simulink model "simulation__"  (R2021a)
settings: Solver=ode14x  StartTime=0.0  StopTime=40  FixedStep=0.01  RelTol=1e-3
values from neighbouring files (symbols this model uses):
  Rep = 1.655    [coefficients.m]
  Rev = 0.04    [coefficients.m]
  Rla = 2.5e-3    (= 0.0025)    [coefficients.m]
  Rpa = 0.023    [coefficients.m]
  Rpp = 0.091    [coefficients.m]
  Rpv = 0.0056    [coefficients.m]
  Rra = 2.5e-3    (= 0.0025)    [coefficients.m]
  Rsa = 0.06    [coefficients.m]
  Rsp = 2.491    [coefficients.m]
  Rsv = 0.038    [coefficients.m]
  Vulv = 16.77    [coefficients.m]
  Vurv = 40.8    [coefficients.m]
libraries: ee_lib x26, fl_lib x20, nesl_utility x11
settings Model: Creator=Buyson  LastModifiedBy=Buyson

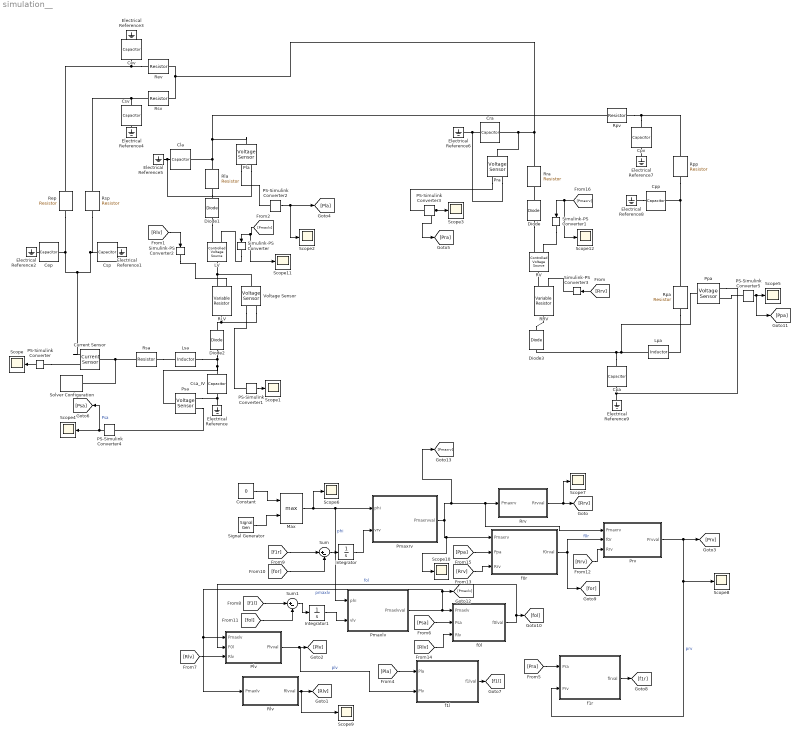
== system simulation__ ==
  Cep : ee_lib/Passive/Capacitor  cap_option=0  c=Cep F  Cvec=[1e-05, 1e-06] F  Vvec=[0, 10] V  CV_table_symmetry=1  f_vec=[1, 10] kHz  DFext_vec=[.8, 1.2]  C_tol=5  enable_C_tol=0  tol_distribution=1  nSigma=4  r=1e-6 Ohm  g=0 1/Ohm  averaging_period=0 s  enable_operating_limits=0  operating_limit_action=2  max_working_voltage_range=[-25, 25] V  power_rating=1 W  enable_faults=0  fault_action=1  Cscale_faulted=100  R_faulted=1e-3 Ohm  G_faulted=0 1/Ohm  tau_fault=1e-3 s  enable_temporal_fault=0  t_fault=1 s  enable_behavioral_fault=0  max_permissible_voltage_range=[-100, 100] V  t_fail_on_voltage=1 s  i_specify=off  i_priority=None  i=0 A  i_nominal_specify=off  i_nominal_unit=A  i_nominal_value=1  v_specify=off  v_priority=None  v=0 V  v_nominal_specify=off  v_nominal_unit=V  v_nominal_value=1  vc_specify=on  vc_priority=High  vc=Cep_IV V  vc_nominal_specify=off  vc_nominal_unit=V  vc_nominal_value=1
  Cev : ee_lib/Passive/Capacitor  cap_option=0  c=Cev F  Cvec=[1e-05, 1e-06] F  Vvec=[0, 10] V  CV_table_symmetry=1  f_vec=[1, 10] kHz  DFext_vec=[.8, 1.2]  C_tol=5  enable_C_tol=0  tol_distribution=1  nSigma=4  r=1e-6 Ohm  g=0 1/Ohm  averaging_period=0 s  enable_operating_limits=0  operating_limit_action=2  max_working_voltage_range=[-25, 25] V  power_rating=1 W  enable_faults=0  fault_action=1  Cscale_faulted=100  R_faulted=1e-3 Ohm  G_faulted=0 1/Ohm  tau_fault=1e-3 s  enable_temporal_fault=0  t_fault=1 s  enable_behavioral_fault=0  max_permissible_voltage_range=[-100, 100] V  t_fail_on_voltage=1 s  i_specify=off  i_priority=None  i=0 A  i_nominal_specify=off  i_nominal_unit=A  i_nominal_value=1  v_specify=off  v_priority=None  v=0 V  v_nominal_specify=off  v_nominal_unit=V  v_nominal_value=1  vc_specify=on  vc_priority=High  vc=Cev_IV V  vc_nominal_specify=off  vc_nominal_unit=V  vc_nominal_value=1
  Cla : ee_lib/Passive/Capacitor  cap_option=0  c=Cla F  Cvec=[1e-05, 1e-06] F  Vvec=[0, 10] V  CV_table_symmetry=1  f_vec=[1, 10] kHz  DFext_vec=[.8, 1.2]  C_tol=5  enable_C_tol=0  tol_distribution=1  nSigma=4  r=1e-6 Ohm  g=0 1/Ohm  averaging_period=0 s  enable_operating_limits=0  operating_limit_action=2  max_working_voltage_range=[-25, 25] V  power_rating=1 W  enable_faults=0  fault_action=1  Cscale_faulted=100  R_faulted=1e-3 Ohm  G_faulted=0 1/Ohm  tau_fault=1e-3 s  enable_temporal_fault=0  t_fault=1 s  enable_behavioral_fault=0  max_permissible_voltage_range=[-100, 100] V  t_fail_on_voltage=1 s  i_specify=off  i_priority=None  i=0 A  i_nominal_specify=off  i_nominal_unit=A  i_nominal_value=1  v_specify=off  v_priority=None  v=0 V  v_nominal_specify=off  v_nominal_unit=V  v_nominal_value=1  vc_specify=on  vc_priority=High  vc=Cla_IV V  vc_nominal_specify=off  vc_nominal_unit=V  vc_nominal_value=1
  Constant : Constant  Value=0
  Cpa : ee_lib/Passive/Capacitor  cap_option=0  c=Cpa F  Cvec=[1e-05, 1e-06] F  Vvec=[0, 10] V  CV_table_symmetry=1  f_vec=[1, 10] kHz  DFext_vec=[.8, 1.2]  C_tol=5  enable_C_tol=0  tol_distribution=1  nSigma=4  r=1e-6 Ohm  g=0 1/Ohm  averaging_period=0 s  enable_operating_limits=0  operating_limit_action=2  max_working_voltage_range=[-25, 25] V  power_rating=1 W  enable_faults=0  fault_action=1  Cscale_faulted=100  R_faulted=1e-3 Ohm  G_faulted=0 1/Ohm  tau_fault=1e-3 s  enable_temporal_fault=0  t_fault=1 s  enable_behavioral_fault=0  max_permissible_voltage_range=[-100, 100] V  t_fail_on_voltage=1 s  i_specify=off  i_priority=None  i=0 A  i_nominal_specify=off  i_nominal_unit=A  i_nominal_value=1  v_specify=off  v_priority=None  v=0 V  v_nominal_specify=off  v_nominal_unit=V  v_nominal_value=1  vc_specify=on  vc_priority=High  vc=Cpa_IV V  vc_nominal_specify=off  vc_nominal_unit=V  vc_nominal_value=1
  Cpp : ee_lib/Passive/Capacitor  cap_option=0  c=Cpp F  Cvec=[1e-05, 1e-06] F  Vvec=[0, 10] V  CV_table_symmetry=1  f_vec=[1, 10] kHz  DFext_vec=[.8, 1.2]  C_tol=5  enable_C_tol=0  tol_distribution=1  nSigma=4  r=1e-6 Ohm  g=0 1/Ohm  averaging_period=0 s  enable_operating_limits=0  operating_limit_action=2  max_working_voltage_range=[-25, 25] V  power_rating=1 W  enable_faults=0  fault_action=1  Cscale_faulted=100  R_faulted=1e-3 Ohm  G_faulted=0 1/Ohm  tau_fault=1e-3 s  enable_temporal_fault=0  t_fault=1 s  enable_behavioral_fault=0  max_permissible_voltage_range=[-100, 100] V  t_fail_on_voltage=1 s  i_specify=off  i_priority=None  i=0 A  i_nominal_specify=off  i_nominal_unit=A  i_nominal_value=1  v_specify=off  v_priority=None  v=0 V  v_nominal_specify=off  v_nominal_unit=V  v_nominal_value=1  vc_specify=on  vc_priority=High  vc=Cpp_IV V  vc_nominal_specify=off  vc_nominal_unit=V  vc_nominal_value=1
  Cpv : ee_lib/Passive/Capacitor  cap_option=0  c=Cpv F  Cvec=[1e-05, 1e-06] F  Vvec=[0, 10] V  CV_table_symmetry=1  f_vec=[1, 10] kHz  DFext_vec=[.8, 1.2]  C_tol=5  enable_C_tol=0  tol_distribution=1  nSigma=4  r=1e-6 Ohm  g=0 1/Ohm  averaging_period=0 s  enable_operating_limits=0  operating_limit_action=2  max_working_voltage_range=[-25, 25] V  power_rating=1 W  enable_faults=0  fault_action=1  Cscale_faulted=100  R_faulted=1e-3 Ohm  G_faulted=0 1/Ohm  tau_fault=1e-3 s  enable_temporal_fault=0  t_fault=1 s  enable_behavioral_fault=0  max_permissible_voltage_range=[-100, 100] V  t_fail_on_voltage=1 s  i_specify=off  i_priority=None  i=0 A  i_nominal_specify=off  i_nominal_unit=A  i_nominal_value=1  v_specify=off  v_priority=None  v=0 V  v_nominal_specify=off  v_nominal_unit=V  v_nominal_value=1  vc_specify=on  vc_priority=High  vc=Cpv_IV V  vc_nominal_specify=off  vc_nominal_unit=V  vc_nominal_value=1
  Cra : ee_lib/Passive/Capacitor  cap_option=0  c=Cra F  Cvec=[1e-05, 1e-06] F  Vvec=[0, 10] V  CV_table_symmetry=1  f_vec=[1, 10] kHz  DFext_vec=[.8, 1.2]  C_tol=5  enable_C_tol=0  tol_distribution=1  nSigma=4  r=1e-6 Ohm  g=0 1/Ohm  averaging_period=0 s  enable_operating_limits=0  operating_limit_action=2  max_working_voltage_range=[-25, 25] V  power_rating=1 W  enable_faults=0  fault_action=1  Cscale_faulted=100  R_faulted=1e-3 Ohm  G_faulted=0 1/Ohm  tau_fault=1e-3 s  enable_temporal_fault=0  t_fault=1 s  enable_behavioral_fault=0  max_permissible_voltage_range=[-100, 100] V  t_fail_on_voltage=1 s  i_specify=off  i_priority=None  i=0 A  i_nominal_specify=off  i_nominal_unit=A  i_nominal_value=1  v_specify=off  v_priority=None  v=0 V  v_nominal_specify=off  v_nominal_unit=V  v_nominal_value=1  vc_specify=on  vc_priority=High  vc=Cra_IV V  vc_nominal_specify=off  vc_nominal_unit=V  vc_nominal_value=1
  Csa_IV : ee_lib/Passive/Capacitor  cap_option=0  c=Csa F  Cvec=[1e-05, 1e-06] F  Vvec=[0, 10] V  CV_table_symmetry=1  f_vec=[1, 10] kHz  DFext_vec=[.8, 1.2]  C_tol=5  enable_C_tol=0  tol_distribution=1  nSigma=4  r=1e-6 Ohm  g=0 1/Ohm  averaging_period=0 s  enable_operating_limits=0  operating_limit_action=2  max_working_voltage_range=[-25, 25] V  power_rating=1 W  enable_faults=0  fault_action=1  Cscale_faulted=100  R_faulted=1e-3 Ohm  G_faulted=0 1/Ohm  tau_fault=1e-3 s  enable_temporal_fault=0  t_fault=1 s  enable_behavioral_fault=0  max_permissible_voltage_range=[-100, 100] V  t_fail_on_voltage=1 s  i_specify=off  i_priority=None  i=0 A  i_nominal_specify=off  i_nominal_unit=A  i_nominal_value=1  v_specify=off  v_priority=None  v=0 V  v_nominal_specify=off  v_nominal_unit=V  v_nominal_value=1  vc_specify=on  vc_priority=High  vc=Csa_IV V  vc_nominal_specify=off  vc_nominal_unit=V  vc_nominal_value=1
  Csp : ee_lib/Passive/Capacitor  cap_option=0  c=Csp F  Cvec=[1e-05, 1e-06] F  Vvec=[0, 10] V  CV_table_symmetry=1  f_vec=[1, 10] kHz  DFext_vec=[.8, 1.2]  C_tol=5  enable_C_tol=0  tol_distribution=1  nSigma=4  r=1e-6 Ohm  g=0 1/Ohm  averaging_period=0 s  enable_operating_limits=0  operating_limit_action=2  max_working_voltage_range=[-25, 25] V  power_rating=1 W  enable_faults=0  fault_action=1  Cscale_faulted=100  R_faulted=1e-3 Ohm  G_faulted=0 1/Ohm  tau_fault=1e-3 s  enable_temporal_fault=0  t_fault=1 s  enable_behavioral_fault=0  max_permissible_voltage_range=[-100, 100] V  t_fail_on_voltage=1 s  i_specify=off  i_priority=None  i=0 A  i_nominal_specify=off  i_nominal_unit=A  i_nominal_value=1  v_specify=off  v_priority=None  v=0 V  v_nominal_specify=off  v_nominal_unit=V  v_nominal_value=1  vc_specify=on  vc_priority=High  vc=Csp_IV V  vc_nominal_specify=off  vc_nominal_unit=V  vc_nominal_value=1
  Csv : ee_lib/Passive/Capacitor  cap_option=0  c=Csv F  Cvec=[1e-05, 1e-06] F  Vvec=[0, 10] V  CV_table_symmetry=1  f_vec=[1, 10] kHz  DFext_vec=[.8, 1.2]  C_tol=5  enable_C_tol=0  tol_distribution=1  nSigma=4  r=1e-6 Ohm  g=0 1/Ohm  averaging_period=0 s  enable_operating_limits=0  operating_limit_action=2  max_working_voltage_range=[-25, 25] V  power_rating=1 W  enable_faults=0  fault_action=1  Cscale_faulted=100  R_faulted=1e-3 Ohm  G_faulted=0 1/Ohm  tau_fault=1e-3 s  enable_temporal_fault=0  t_fault=1 s  enable_behavioral_fault=0  max_permissible_voltage_range=[-100, 100] V  t_fail_on_voltage=1 s  i_specify=off  i_priority=None  i=0 A  i_nominal_specify=off  i_nominal_unit=A  i_nominal_value=1  v_specify=off  v_priority=None  v=0 V  v_nominal_specify=off  v_nominal_unit=V  v_nominal_value=1  vc_specify=on  vc_priority=High  vc=Csv_IV V  vc_nominal_specify=off  vc_nominal_unit=V  vc_nominal_value=1
  Current Sensor : fl_lib/Electrical/Electrical Sensors/Current Sensor
  Diode{,1..3} (4 alike) : ee_lib/Semiconductors & Converters/Diode  ModelType=ee.enum.diode.modelType.pwl  IfMat=[.07, .12, .19, 1.75, 4.24, 7.32, 11.2; .16, .3, .72, 2.14, 4.02, 6.35, 9.12] A  TjVec=[25, 125] degC  VfVec=[.5, .7, .9, 1.3, 1.7, 2.1, 2.5] V  Vf=1e-4 V  Ron=1e-10 Ohm  Goff=1e-10 S  prmExp=ee.enum.diode.expParam.useTwo  I12=[.0137, .545] A  V12=[.6, .7] V  IS=1e-12 A  ec=1  I1=0.0137 A  V1=0.6 V  RS=0 Ohm  Tmeas=25 degC  N_series=1  N_parallel=1  Rz=0.3 Ohm  BV=inf V  C_param=ee.enum.diode.capParam.fixed  CJ=5 pF  CJ0=5 pF  VJ=1 V  Mgrad=0.5  Vvec=[.1, 10, 100] V  Cvec=[3.5, 1, .4] pF  FC=0.5  Q_param=ee.enum.diode.recoveryParam.off  iRM=-7.15 A  iF=4 A  didt=-750 A/us  trr_factor=3  trr=115 ns  Qrr=150 s*nA  TT=50 ns  tau=100 ns  T_param=ee.enum.diode.temperatureParam.off  IS_T2=1.25e-7 A  I1_T2=0.245 A  V1_T2=0.5 V  Tmeas2=125 degC  EG_param=ee.enum.diode.egapParam.material_si  EG=1.11 eV  XTI_param=ee.enum.diode.xtiParam.pn  XTI=3  dBVdT=0 V/K  enable_faults=ee.enum.faults.faultEnable.no  fault_action=ee.enum.faults.faultAction.none  fault_types=ee.enum.diode.faults.open  tau_fault=1e-3 s  IfMat_faulted=[.07, .12, .19, 1.75, 4.24, 7.32, 11.2; .16, .3, .72, 2.14, 4.02, 6.35, 9.12] A  VfVec_faulted=[.5, .7, .9, 1.3, 1.7, 2.1, 2.5] V  Ropen_faulted=1000 Ohm  Gshort_faulted=1000 1/Ohm  Vf_faulted=0.6 V  Ron_faulted=0.3 Ohm  Goff_faulted=1e-8 S  I12_faulted=[.0137, .545] A  V12_faulted=[.6, .7] V  IS_faulted=1e-12 A  ec_faulted=1  I1_faulted=0.0137 A  V1_faulted=0.6 V  RS_faulted=0 Ohm  Rz_faulted=0.3 Ohm  BV_faulted=inf V  Cscale_faulted=100  enable_temporal_fault=ee.enum.faults.faultEnable.no  t_fault=inf s  enable_behavioral_fault=ee.enum.faults.faultEnable.no  max_permissible_voltage=inf V  n_fail_on_voltage=1  max_permissible_current=inf A  t_fail_on_current=1 s  max_permissible_dVdt=inf V/s  Tdevice=25 degC  i_specify=off  i_priority=None  i=0 A  i_nominal_specify=off  i_nominal_unit=A  i_nominal_value=1  v_specify=on  v_priority=None  v=1e-4 V  v_nominal_specify=off  v_nominal_unit=V  v_nominal_value=1  i_diode_specify=off  i_diode_priority=None  i_diode=0 A  i_diode_nominal_specify=off  i_diode_nominal_unit=A  i_diode_nominal_value=1  v_diode_specify=off  v_diode_priority=None  v_diode=0 V  v_diode_nominal_specify=off  v_diode_nominal_unit=V  v_diode_nominal_value=1  i_capacitor_specify=off  i_capacitor_priority=None  i_capacitor=0 A  i_capacitor_nominal_specify=off  i_capacitor_nominal_unit=A  i_capacitor_nominal_value=1  v_capacitor_specify=off  v_capacitor_priority=None  v_capacitor=0 V  v_capacitor_nominal_specify=off  v_capacitor_nominal_unit=V  v_capacitor_nominal_value=1  power_dissipated_specify=off  power_dissipated_priority=None  power_dissipated=0 W  power_dissipated_nominal_specify=off  power_dissipated_nominal_unit=W  power_dissipated_nominal_value=1  max_permissible_temperature=inf K  t_fail_on_temperature=1 s  thermal_network_parameterization=ee.enum.thermalNetworkTopology.cauer  Rth=[0, 10] K/W  Rth_Foster=[4, 6] K/W  thermal_mass_parameterization=ee.enum.thermalNetwork.timeconstant  thermal_mass=[0, 1] J/K  thermal_mass_Foster=[1.5, 3] J/K  thermal_time_constant=[0, 10] s  thermal_time_constant_Foster=[6, 18] s  thermal_mass_initial_temperatures=[25, 25] degC
  Electrical Reference{,1..9} (10 alike) : fl_lib/Electrical/Electrical Elements/Electrical Reference
  Integrator : Integrator  InitialCondition=Vurv
  Integrator1 : Integrator  InitialCondition=Vulv
  LV : fl_lib/Electrical/Electrical Sources/Controlled Voltage Source
  Lpa : ee_lib/Passive/Inductor  l=Lpa H  L_tol=20  enable_L_tol=0  tol_distribution=1  nSigma=4  r=0 Ohm  g=1e-9 1/Ohm  enable_operating_limits=0  operating_limit_action=2  max_working_current=1 A  power_rating=1 W  enable_faults=0  fault_action=1  lambdaPercent=50  k_faulted=0.9999  turnsShort=0  openCct=0  groundShort=0  groundShortG=0 1/Ohm  tau_fault=1e-3 s  enable_temporal_fault=0  t_fault=1 s  enable_behavioral_fault=0  max_permissible_voltage=100 V  n_fail_on_voltage=1  max_permissible_current=1 A  t_fail_on_current=1 s  i_L_specify=off  i_L_priority=High  i_L=0 A  i_L_nominal_specify=off  i_L_nominal_unit=A  i_L_nominal_value=1
  Lsa : ee_lib/Passive/Inductor  l=Lsa H  L_tol=20  enable_L_tol=0  tol_distribution=1  nSigma=4  r=0 Ohm  g=1e-9 1/Ohm  enable_operating_limits=0  operating_limit_action=2  max_working_current=1 A  power_rating=1 W  enable_faults=0  fault_action=1  lambdaPercent=50  k_faulted=0.9999  turnsShort=0  openCct=0  groundShort=0  groundShortG=0 1/Ohm  tau_fault=1e-3 s  enable_temporal_fault=0  t_fault=1 s  enable_behavioral_fault=0  max_permissible_voltage=100 V  n_fail_on_voltage=1  max_permissible_current=1 A  t_fail_on_current=1 s  i_L_specify=off  i_L_priority=High  i_L=0 A  i_L_nominal_specify=off  i_L_nominal_unit=A  i_L_nominal_value=1
  Max : MinMax  Function=max  Inputs=2
  PS-Simulink Converter{,1..5} (6 alike) : nesl_utility/PS-Simulink Converter  PhysicalDomain=network_engine_domain  SubClassName=ps_output  LeftPortType=input  RightPortType=output  PseudoPeriodic=off  Frequencies=[]  Unit=inherit  AffineConversion=off
      settings: SourceProductBaseCode=PW,SS
  Pla : fl_lib/Electrical/Electrical Sensors/Voltage Sensor
  Plv : MATLAB Function  TreatAsAtomicUnit=on
  Pmaxlv : MATLAB Function  TreatAsAtomicUnit=on
  Pmaxrv : MATLAB Function  TreatAsAtomicUnit=on
  Ppa : fl_lib/Electrical/Electrical Sensors/Voltage Sensor
  Pra : fl_lib/Electrical/Electrical Sensors/Voltage Sensor
  Prv : MATLAB Function  TreatAsAtomicUnit=on
  Psa : fl_lib/Electrical/Electrical Sensors/Voltage Sensor
  RLV : fl_lib/Electrical/Electrical Elements/Variable Resistor  Rmin=0 Ohm  i_specify=off  i_priority=None  i=0 A  i_nominal_specify=off  i_nominal_unit=A  i_nominal_value=1  v_specify=off  v_priority=None  v=0 V  v_nominal_specify=off  v_nominal_unit=V  v_nominal_value=1
  RRV : fl_lib/Electrical/Electrical Elements/Variable Resistor  Rmin=0 Ohm  i_specify=off  i_priority=None  i=0 A  i_nominal_specify=off  i_nominal_unit=A  i_nominal_value=1  v_specify=off  v_priority=None  v=0 V  v_nominal_specify=off  v_nominal_unit=V  v_nominal_value=1
  RV : fl_lib/Electrical/Electrical Sources/Controlled Voltage Source
  Rep : ee_lib/Passive/Resistor  R=Rep Ohm  R_tol=5  enable_R_tol=0  tol_distribution=1  nSigma=4  enable_operating_limits=0  operating_limit_action=2  max_working_voltage=100 V  power_rating=1 W  enable_faults=0  fault_action=1  R_faulted=inf Ohm  enable_temporal_fault=0  t_fault=1 s  enable_behavioral_fault=0  max_permissible_current=1 A  t_fail_on_current=1 s  noise_mode=0  sample_time=1e-3 s  repeatability=1  auto_seed=3499211588  user_seed=0  Tdevice=25 degC  alpha=3.93e-3 1/K  Tmeas=25 degC  thermal_mass=100 J/K  power_derating_T1=70 degC  power_derating_T2=155 degC  operating_temperature_range_vec=[-50, 150] degC  temperature_specify=off  temperature_priority=High  temperature=298.15 K  temperature_nominal_specify=off  temperature_nominal_unit=K  temperature_nominal_value=1
  Rev : ee_lib/Passive/Resistor  R=Rev Ohm  R_tol=5  enable_R_tol=0  tol_distribution=1  nSigma=4  enable_operating_limits=0  operating_limit_action=2  max_working_voltage=100 V  power_rating=1 W  enable_faults=0  fault_action=1  R_faulted=inf Ohm  enable_temporal_fault=0  t_fault=1 s  enable_behavioral_fault=0  max_permissible_current=1 A  t_fail_on_current=1 s  noise_mode=0  sample_time=1e-3 s  repeatability=1  auto_seed=3890346746  user_seed=0  Tdevice=25 degC  alpha=3.93e-3 1/K  Tmeas=25 degC  thermal_mass=100 J/K  power_derating_T1=70 degC  power_derating_T2=155 degC  operating_temperature_range_vec=[-50, 150] degC  temperature_specify=off  temperature_priority=High  temperature=298.15 K  temperature_nominal_specify=off  temperature_nominal_unit=K  temperature_nominal_value=1
  Rla : ee_lib/Passive/Resistor  R=Rla Ohm  R_tol=5  enable_R_tol=0  tol_distribution=1  nSigma=4  enable_operating_limits=0  operating_limit_action=2  max_working_voltage=100 V  power_rating=1 W  enable_faults=0  fault_action=1  R_faulted=inf Ohm  enable_temporal_fault=0  t_fault=1 s  enable_behavioral_fault=0  max_permissible_current=1 A  t_fail_on_current=1 s  noise_mode=0  sample_time=1e-3 s  repeatability=1  auto_seed=545404223  user_seed=0  Tdevice=25 degC  alpha=3.93e-3 1/K  Tmeas=25 degC  thermal_mass=100 J/K  power_derating_T1=70 degC  power_derating_T2=155 degC  operating_temperature_range_vec=[-50, 150] degC  temperature_specify=off  temperature_priority=High  temperature=298.15 K  temperature_nominal_specify=off  temperature_nominal_unit=K  temperature_nominal_value=1
  Rlv : MATLAB Function  TreatAsAtomicUnit=on
  Rpa : ee_lib/Passive/Resistor  R=Rpa Ohm  R_tol=5  enable_R_tol=0  tol_distribution=1  nSigma=4  enable_operating_limits=0  operating_limit_action=2  max_working_voltage=100 V  power_rating=1 W  enable_faults=0  fault_action=1  R_faulted=inf Ohm  enable_temporal_fault=0  t_fault=1 s  enable_behavioral_fault=0  max_permissible_current=1 A  t_fail_on_current=1 s  noise_mode=0  sample_time=1e-3 s  repeatability=1  auto_seed=3922919431  user_seed=0  Tdevice=25 degC  alpha=3.93e-3 1/K  Tmeas=25 degC  thermal_mass=100 J/K  power_derating_T1=70 degC  power_derating_T2=155 degC  operating_temperature_range_vec=[-50, 150] degC  temperature_specify=off  temperature_priority=High  temperature=298.15 K  temperature_nominal_specify=off  temperature_nominal_unit=K  temperature_nominal_value=1
  Rpp : ee_lib/Passive/Resistor  R=Rpp Ohm  R_tol=5  enable_R_tol=0  tol_distribution=1  nSigma=4  enable_operating_limits=0  operating_limit_action=2  max_working_voltage=100 V  power_rating=1 W  enable_faults=0  fault_action=1  R_faulted=inf Ohm  enable_temporal_fault=0  t_fault=1 s  enable_behavioral_fault=0  max_permissible_current=1 A  t_fail_on_current=1 s  noise_mode=0  sample_time=1e-3 s  repeatability=1  auto_seed=2715962282  user_seed=0  Tdevice=25 degC  alpha=3.93e-3 1/K  Tmeas=25 degC  thermal_mass=100 J/K  power_derating_T1=70 degC  power_derating_T2=155 degC  operating_temperature_range_vec=[-50, 150] degC  temperature_specify=off  temperature_priority=High  temperature=298.15 K  temperature_nominal_specify=off  temperature_nominal_unit=K  temperature_nominal_value=1
  Rpv : ee_lib/Passive/Resistor  R=Rpv Ohm  R_tol=5  enable_R_tol=0  tol_distribution=1  nSigma=4  enable_operating_limits=0  operating_limit_action=2  max_working_voltage=100 V  power_rating=1 W  enable_faults=0  fault_action=1  R_faulted=inf Ohm  enable_temporal_fault=0  t_fault=1 s  enable_behavioral_fault=0  max_permissible_current=1 A  t_fail_on_current=1 s  noise_mode=0  sample_time=1e-3 s  repeatability=1  auto_seed=418932850  user_seed=0  Tdevice=25 degC  alpha=3.93e-3 1/K  Tmeas=25 degC  thermal_mass=100 J/K  power_derating_T1=70 degC  power_derating_T2=155 degC  operating_temperature_range_vec=[-50, 150] degC  temperature_specify=off  temperature_priority=High  temperature=298.15 K  temperature_nominal_specify=off  temperature_nominal_unit=K  temperature_nominal_value=1
  Rra : ee_lib/Passive/Resistor  R=Rra Ohm  R_tol=5  enable_R_tol=0  tol_distribution=1  nSigma=4  enable_operating_limits=0  operating_limit_action=2  max_working_voltage=100 V  power_rating=1 W  enable_faults=0  fault_action=1  R_faulted=inf Ohm  enable_temporal_fault=0  t_fault=1 s  enable_behavioral_fault=0  max_permissible_current=1 A  t_fail_on_current=1 s  noise_mode=0  sample_time=1e-3 s  repeatability=1  auto_seed=1196140742  user_seed=0  Tdevice=25 degC  alpha=3.93e-3 1/K  Tmeas=25 degC  thermal_mass=100 J/K  power_derating_T1=70 degC  power_derating_T2=155 degC  operating_temperature_range_vec=[-50, 150] degC  temperature_specify=off  temperature_priority=High  temperature=298.15 K  temperature_nominal_specify=off  temperature_nominal_unit=K  temperature_nominal_value=1
  Rrv : MATLAB Function  TreatAsAtomicUnit=on
  Rsa : ee_lib/Passive/Resistor  R=Rsa Ohm  R_tol=5  enable_R_tol=0  tol_distribution=1  nSigma=4  enable_operating_limits=0  operating_limit_action=2  max_working_voltage=100 V  power_rating=1 W  enable_faults=0  fault_action=1  R_faulted=inf Ohm  enable_temporal_fault=0  t_fault=1 s  enable_behavioral_fault=0  max_permissible_current=1 A  t_fail_on_current=1 s  noise_mode=0  sample_time=1e-3 s  repeatability=1  auto_seed=2348838240  user_seed=0  Tdevice=25 degC  alpha=3.93e-3 1/K  Tmeas=25 degC  thermal_mass=100 J/K  power_derating_T1=70 degC  power_derating_T2=155 degC  operating_temperature_range_vec=[-50, 150] degC  temperature_specify=off  temperature_priority=High  temperature=298.15 K  temperature_nominal_specify=off  temperature_nominal_unit=K  temperature_nominal_value=1
  Rsp : ee_lib/Passive/Resistor  R=Rsp Ohm  R_tol=5  enable_R_tol=0  tol_distribution=1  nSigma=4  enable_operating_limits=0  operating_limit_action=2  max_working_voltage=100 V  power_rating=1 W  enable_faults=0  fault_action=1  R_faulted=inf Ohm  enable_temporal_fault=0  t_fault=1 s  enable_behavioral_fault=0  max_permissible_current=1 A  t_fail_on_current=1 s  noise_mode=0  sample_time=1e-3 s  repeatability=1  auto_seed=4112460543  user_seed=0  Tdevice=25 degC  alpha=3.93e-3 1/K  Tmeas=25 degC  thermal_mass=100 J/K  power_derating_T1=70 degC  power_derating_T2=155 degC  operating_temperature_range_vec=[-50, 150] degC  temperature_specify=off  temperature_priority=High  temperature=298.15 K  temperature_nominal_specify=off  temperature_nominal_unit=K  temperature_nominal_value=1
  Rsv : ee_lib/Passive/Resistor  R=Rsv Ohm  R_tol=5  enable_R_tol=0  tol_distribution=1  nSigma=4  enable_operating_limits=0  operating_limit_action=2  max_working_voltage=100 V  power_rating=1 W  enable_faults=0  fault_action=1  R_faulted=inf Ohm  enable_temporal_fault=0  t_fault=1 s  enable_behavioral_fault=0  max_permissible_current=1 A  t_fail_on_current=1 s  noise_mode=0  sample_time=1e-3 s  repeatability=1  auto_seed=4144164703  user_seed=0  Tdevice=25 degC  alpha=3.93e-3 1/K  Tmeas=25 degC  thermal_mass=100 J/K  power_derating_T1=70 degC  power_derating_T2=155 degC  operating_temperature_range_vec=[-50, 150] degC  temperature_specify=off  temperature_priority=High  temperature=298.15 K  temperature_nominal_specify=off  temperature_nominal_unit=K  temperature_nominal_value=1
  Scope{,1..12} (13 alike) : Scope
  Signal Generator : SignalGenerator  Frequency=8  Units=rad/sec
  Simulink-PS Converter{,1..3} (4 alike) : nesl_utility/Simulink-PS Converter  PhysicalDomain=network_engine_domain  SubClassName=ps_input  LeftPortType=input  RightPortType=output  PseudoPeriodic=off  Frequencies=[]  NoiseDistribution=none  NoiseParameters=[]  Unit=1  AffineConversion=off  FilteringAndDerivatives=provide  SimscapeFilterOrder=1  InputFilterTimeConstant=0.001  UdotUserProvided=0
      settings: SourceProductBaseCode=PW,SS
  Solver Configuration : nesl_utility/Solver Configuration  PhysicalDomain=network_engine_domain  SubClassName=solver  LeftPortType=input  RightPortType=generic  Tones=[]  Harmonics=[]  SimulateNoise=off  Profile=off  UseLocalSampling=off  EnableSwitchedLinearOptims=on  FrequencyDomain=off  UseCCode=off  RelTol=0.001  AbsTol=1e-06  MinStep=1e-09  ToWorkspace=off  RevertToSquareIcSolve=off  NumHomotopyIterations=100  PhasorMode=off  PhasorModeNumHarmonics=1  DoDC=off  ResidualTolerance=1e-09  UseLocalSolver=off  LocalSolverChoice=NE_BACKWARD_EULER_ADVANCER  LocalSolverSampleTime=0.001  DoFixedCost=off  MaxNonlinIter=3  MaxModeIter=2  ComputeImpulses=off  ImpulseIterations=2  LinearAlgebra=auto  EquationFormulation=NE_TIME_EF  DelaysMemoryBudget=1024  AutomaticFiltering=on  FilteringTimeConstant=0.001  PartitionStorageMethod=AS_NEEDED  PartitionMemoryBudget=1024  PartitionMethod=ROBUST
      settings: SourceProductBaseCode=PW,SS
  Sum : Sum  Inputs=|+-
  Sum1 : Sum  Inputs=|+-
  Voltage Sensor : fl_lib/Electrical/Electrical Sensors/Voltage Sensor
  f0l : MATLAB Function  TreatAsAtomicUnit=on
  f0r : MATLAB Function  TreatAsAtomicUnit=on
  f1l : MATLAB Function  TreatAsAtomicUnit=on
  f1r : MATLAB Function  TreatAsAtomicUnit=on
  wires:
  [Ppa] -> f0r/2(Ppa)
  Signal Generator/1 -> Max/2
  f0r/1(f0rval) -> [for], Prv/2(f0r)  "f0r"
  [Rrv] -> Simulink-PS Converter3/1
  Pmaxrv/1(Pmaxrvval) -> Scope10/1, f0r/1(Pmaxrv), [Pmaxrv], Prv/1(Pmaxrv), Rrv/1(Pmaxrv)
  PS-Simulink Converter5/1 -> [Ppa], Scope5/1
  [Rrv] -> Prv/3(Rrv)
  PS-Simulink Converter2/1 -> [Pla], Scope2/1
  [Rlv] -> Plv/3(Rlv)
  [Rrv] -> f0r/3(Rrv)
  Max/1 -> Scope6/1, Pmaxlv/1(phi), Pmaxrv/1(phi)  "phi"
  [Rlv] -> f0l/3(Rlv)
  Plv/1(Plvval) -> f1l/2(Plv), [Plv]  "plv"
  [f1l] -> Sum1/1
  [fol] -> Sum1/2
  f1l/1(f1lval) -> [f1l]
  PS-Simulink Converter1/1 -> Scope1/1
  Integrator1/1 -> Pmaxlv/2(vlv)
  PS-Simulink Converter3/1 -> Scope3/1, [Pra]
  [Pla] -> f1l/1(Pla)
  Integrator/1 -> Pmaxrv/2(vrv)
  Sum1/1 -> Integrator1/1
  Rlv/1(Rlvval) -> Scope9/1, [Rlv]
  [Psa] -> f0l/2(Psa)
  [f1r] -> Sum/1
  [for] -> Sum/2
  [Pra] -> f1r/1(Pra)
  f1r/1(flrval) -> [f1r]
  PS-Simulink Converter4/1 -> [Psa], Scope4/1  "Psa"
  Prv/1(Prvval) -> f1r/2(Prv), Scope8/1, [Prv]  "prv"
  [Pmaxlv] -> Scope11/1, Simulink-PS Converter/1
  Sum/1 -> Integrator/1
  PS-Simulink Converter/1 -> Scope/1
  Rrv/1(Rrvval) -> Scope7/1, [Rrv]
  Pmaxlv/1(Pmaxlvval) -> Rlv/1(Pmaxlv), Plv/1(Pmaxlv), [Pmaxlv], f0l/1(Pmaxlv)  "pmaxlv"
  [Rlv] -> Simulink-PS Converter2/1
  Constant/1 -> Max/1
  f0l/1(f0lval) -> [fol], Plv/2(F0l)  "fol"
  [Pmaxrv] -> Scope12/1, Simulink-PS Converter1/1
  connections:
  Current Sensor/LConn1 -- Rsa/RConn1 -- Solver Configuration/RConn1
  Cpv/LConn1 -- Rpv/RConn1 -- Rpp/LConn1
  Csa_IV/LConn1 -- Diode2/RConn1 -- Lsa/LConn1 -- Psa/LConn1
  Cra/LConn1 -- Rsv/RConn1 -- Rev/RConn1 -- Rra/LConn1 -- Pra/LConn1
  Cpp/LConn1 -- Rpp/RConn1 -- Rpa/LConn1
  Electrical Reference5/LConn1 -- Cla/RConn1 -- Pla/RConn2
  Cpa/RConn1 -- Electrical Reference9/LConn1 -- Ppa/RConn2
  Cpa/LConn1 -- Diode3/RConn1 -- Lpa/RConn1 -- Ppa/LConn1
  Pra/RConn2 -- Cra/RConn1 -- Electrical Reference6/LConn1
  Pla/LConn1 -- Rla/LConn1 -- Cla/LConn1 -- Rpv/LConn1
  Cep/LConn1 -- Rep/LConn1 -- Rsp/LConn1 -- Csp/LConn1 -- Current Sensor/RConn2
  Csv/LConn1 -- Rsp/RConn1 -- Rsv/LConn1
  RLV/LConn2 -- LV/LConn1 -- Voltage Sensor/LConn1
  Rev/LConn1 -- Rep/RConn1 -- Cev/LConn1
  Psa/RConn2 -- Electrical Reference/LConn1 -- Csa_IV/RConn1
  Voltage Sensor/RConn1 -- PS-Simulink Converter1/LConn1
  Electrical Reference1/LConn1 -- Csp/RConn1
  RRV/RConn1 -- Diode3/LConn1
  Diode/RConn1 -- RV/RConn2
  PS-Simulink Converter5/LConn1 -- Ppa/RConn1
  Pra/RConn1 -- PS-Simulink Converter3/LConn1
  Diode/LConn1 -- Rra/RConn1
  Pla/RConn1 -- PS-Simulink Converter2/LConn1
  Simulink-PS Converter2/RConn1 -- RLV/LConn1
  Diode1/RConn1 -- LV/RConn2
  Diode2/LConn1 -- Voltage Sensor/RConn2 -- RLV/RConn1
  Rla/RConn1 -- Diode1/LConn1
  Simulink-PS Converter3/RConn1 -- RRV/LConn1
  Simulink-PS Converter1/RConn1 -- RV/RConn1
  Electrical Reference7/LConn1 -- Cpv/RConn1
  Electrical Reference2/LConn1 -- Cep/RConn1
  Simulink-PS Converter/RConn1 -- LV/RConn1
  Rsa/LConn1 -- Lsa/RConn1
  Electrical Reference4/LConn1 -- Csv/RConn1
  Electrical Reference8/LConn1 -- Cpp/RConn1
  Psa/RConn1 -- PS-Simulink Converter4/LConn1
  RRV/LConn2 -- RV/LConn1
  Electrical Reference3/LConn1 -- Cev/RConn1
  Rpa/RConn1 -- Lpa/LConn1
  PS-Simulink Converter/LConn1 -- Current Sensor/RConn1

== matlab function simulation__/Pmaxrv ==
  data: phi input; Pmaxrvval output; vrv input
function Pmaxrvval = Pmaxrv(phi, vrv)

Vurv = 40.8;
P0rv = 1.5; 
kErv = 0.011;
 Emaxrv0 = 1.75;



Pmaxrvval = phi*Emaxrv0*(vrv - Vurv) + (1 - phi)*P0rv*(exp(kErv*vrv)-1);

end

== matlab function simulation__/Rrv ==
  data: Pmaxrv input; Rrvval output
function Rrvval = Rrv(Pmaxrv)
kRrv = 1.4e-3;

Rrvval = kRrv*Pmaxrv;

end

== matlab function simulation__/Pmaxlv ==
  data: phi input; Pmaxlvval output; vlv input
function Pmaxlvval = Pmaxlv(phi, vlv)
Vulv = 16.77;  
P0lv = 1.5;  
kElv = 0.014;    
Emaxlv0 = 2.95; 

Pmaxlvval = phi*Emaxlv0*(vlv - Vulv) + (1 - phi)*P0lv*(exp(kElv*vlv)-1);

end

== matlab function simulation__/f1r ==
  data: Pra input; flrval output; Prv input
function flrval = flr(Pra, Prv)

   Rra = 2.5e-3;

    if(Pra <= Prv)
        flrval = 0;
    else
        flrval = (Pra - Prv)/Rra;
    end
        
end

== matlab function simulation__/f0l ==
  data: Pmaxlv input; f0lval output; Psa input; Rlv input
function f0lval = f0l(Pmaxlv, Psa, Rlv)

    if(Pmaxlv <= Psa)
        f0lval = 0;
    else
        f0lval = (Pmaxlv - Psa)/Rlv;
    end

end

== matlab function simulation__/Rlv ==
  data: Pmaxlv input; Rlvval output
function Rlvval = Rlv(Pmaxlv)
kRlv = 3.75e-4;

Rlvval = kRlv * Pmaxlv;

end

== matlab function simulation__/Plv ==
  data: Pmaxlv input; Plvval output; F0l input; Rlv input
function Plvval = Plv(Pmaxlv, F0l, Rlv)

Plvval = Pmaxlv - Rlv * F0l;


end

== matlab function simulation__/f1l ==
  data: Pla input; f1lval output; Plv input
function f1lval = f1l(Pla, Plv)

Rla = 2.5e-3;   

if(Pla <= Plv)
    f1lval = 0;
    
else
    f1lval = (Pla - Plv)/(Rla);
    
end
end

== matlab function simulation__/Prv ==
  data: Pmaxrv input; Prvval output; f0r input; Rrv input
function Prvval = Prv(Pmaxrv, f0r, Rrv)

Prvval = Pmaxrv - Rrv*f0r;

end

== matlab function simulation__/f0r ==
  data: Pmaxrv input; f0rval output; Ppa input; Rrv input
function f0rval = f0r(Pmaxrv, Ppa, Rrv)

    if(Pmaxrv <= Ppa)
        f0rval = 0;
    else
        f0rval = (Pmaxrv - Ppa)/Rrv;
    end

end
